simulink model "test3"  (Simulink 7.1)
settings: Solver=ode45  StartTime=0.0  StopTime=10.0  RelTol=1e-3
values from neighbouring files (symbols this model uses):
  Ctorque = cq(2:5:102,2:5:182)    [cq_table.m]
settings Model: Creator=xc  LastModifiedBy=xc

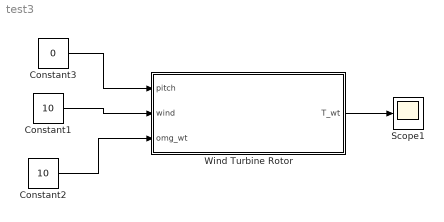
== system test3 ==
  Constant1 : Constant  Value=10  OutDataType=sfix(16)  OutScaling=2^0
  Constant2 : Constant  Value=10  OutDataType=sfix(16)  OutScaling=2^0
  Constant3 : Constant  Value=0  OutDataType=sfix(16)  OutScaling=2^0
  Scope1 : Scope
      settings: YMin=-2.25e+010  YMax=1.5e+010
  Wind Turbine Rotor : Subsystem  AncestorBlock=wt_blockset_beta/Mechanical Components/Wind Turbine Rotor  mask(Aerodynamic model for wind turbine){R=40, ro_air=1.25, cut_in=3, cut_out=25, Tact=1}
      mask prompts: R "Blade radius [m]"; ro_air "Air density [kg m3]"; cut_in "Cut in speed [m/sec]"; cut_out "Cut out speed [m/sec]"; Tact "Time constant for pitch actuator [sec]"
      mask init:
      | cq_table
      mask Display: plot(20,0,120,200,[45,35,35,45,75,75,45],[85,92,108,115,115,85,85],[55,50,70,65],[115,180,190,115],[55,50,70,65],[85,10,20,85],[75,85],[102,102],[75,85],[98,98],[105,85,85,105],[80,85,115,120])
  wires:
  Constant3/1 -> Wind Turbine Rotor/1(pitch)
  Constant1/1 -> Wind Turbine Rotor/2(wind)
  Constant2/1 -> Wind Turbine Rotor/3(omg_wt)
  Wind Turbine Rotor/1(T_wt) -> Scope1/1

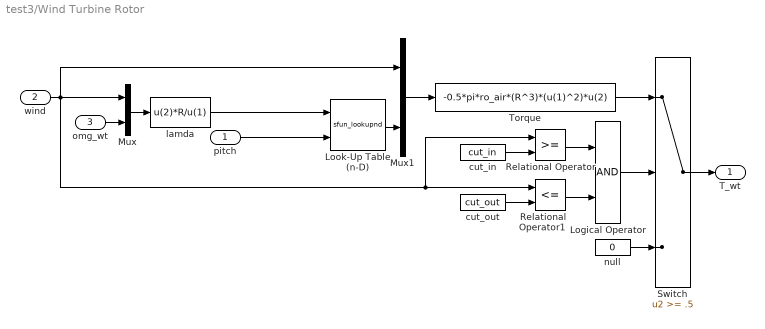
== system test3/Wind Turbine Rotor ==
  pitch : Inport  OutDataType=sfix(16)  OutScaling=2^0
  wind : Inport  Port=2  OutDataType=sfix(16)  OutScaling=2^0
  omg_wt : Inport  Port=3  OutDataType=sfix(16)  OutScaling=2^0
  Logical Operator : Logic
  Look-Up Table (n-D) : S-Function  FunctionName=sfun_lookupnd  Parameters=numDims,tableData,bp1,bp2,bp3,bp4,bpcell,searchMode,cacheBpFlag,vectorInputFlag,interpMethod,extrapMethod,rangeErrorMode  EnableBusSupport=off  mask(LookupNDInterp){numDimsPopupSelect=2, bp1=[0:1:20], bp2=[-90:5:90], bp3=[1:3], bp4=[1:3], bpcell={ [1:3], [1:3] }, explicitNumDims=2, searchMode=Binary Search, cacheBpFlag=off, vectorInputFlag=off, tableData=Ctorque, interpMethod=Linear, extrapMethod=None - Clip, rangeErrorMode=Error}
      mask prompts: numDimsPopupSelect "Number of table dimensions:"; bp1 "First input (row) breakpoint set:"; bp2 "Second (column) input breakpoint set:"; bp3 "Third input breakpoint set:"; bp4 "Fourth input breakpoint set:"; bpcell "Fifth..Nth breakpoint sets (cell array):"; explicitNumDims "Explicit number of dimensions:"; searchMode "Index search method:"; cacheBpFlag "Begin index searches using previous index results"; vectorInputFlag "Use one (vector) input port instead of N ports"; tableData "Table data:"; interpMethod "Interpolation method:"; extrapMethod "Extrapolation method:"; rangeErrorMode "Action for out of range input:"
      mask help: Perform n-dimensional interpolated table lookup including index searches. The table is a sampled representation of a function in N variables. Breakpoint sets relate the input values to positions in the table. The first dimension corresponds to the top (or left) input port.
      mask init:
      | if numDimsPopupSelect==5
      |   numDims=explicitNumDims;
      | else
      |   numDims=numDimsPopupSelect;
      | end
      | if strcmp(get_param(bdroot(gcb),'BlockDiagramType'),'library')
      |   dimsChar = 'n';
      | else
      |   dimsChar = sprintf('%d',numDims);
      | end
      | switch interpMethod
      |   case 1
      |     plottype = 'flatplot';
      |   case 2
      |     plottype = 'lineplot';
      |   otherwise
      |     plottype = 'splineplot';
      | end
      | for i=1:numDims
      |   switch( i )
      |     case 1
      |       bp = bp1;
      |     case 2
      |       bp = bp2;
      |     case 3
      |       bp = bp3;
      |     case 4
      |       bp = bp4;
      |     otherwise
      |       bp = bpcell{i-4};
      |    end
      |    Lbp = length(bp);
      |    if i < 2
      |      bpData = reshape(bp,Lbp,1);
      |      bpIndices = 0;
      |    else
      |      bpData = [ bpData; reshape(bp,Lbp,1) ];
      |      bpIndices = [ bpIndices; bpIndices(i-1)+LbpPrev ];
      |    end
      |    LbpPrev = Lbp;
      | end
      | [x,y,xaxes,yaxes] = ndlookico(plottype, numDims,{bpData,bpIndices,tableData});
      mask StyleString: popup(   1   |   2   |   3   |   4   |More...),edit,edit,edit,edit,edit,edit,popup(Evenly Spaced Points|Linear Search|Binary Search),checkbox,checkbox,edit,popup(None - Flat|Linear|Cubic Spline),popup(None - Clip|Linear|Cubic Spline),popup(None|Warning|Error)
      mask CallbackString: ndlookico|||||||||||||
      mask Display:
      | text(0.5,0.9,sprintf(' %s-D T(u)',dimsChar),'horizontalAlignment','center')
      | plot(x,y)
      | plot(xaxes,yaxes)
  Mux : Mux  Inputs=2
  Mux1 : Mux  Inputs=2
  Relational Operator : RelationalOperator  InputSameDT=on
  Relational Operator1 : RelationalOperator  Operator=<=  InputSameDT=on
  Switch : Switch  Threshold=.5  SaturateOnIntegerOverflow=on  InputSameDT=on
  Torque : Fcn  Expr=-0.5*pi*ro_air*(R^3)*(u(1)^2)*u(2)
  cut_in : Constant  Value=cut_in  OutDataType=sfix(16)  OutScaling=2^0
  cut_out : Constant  Value=cut_out  OutDataType=sfix(16)  OutScaling=2^0
  lamda : Fcn  Expr=u(2)*R/u(1)
  null : Constant  Value=0  OutDataType=sfix(16)  OutScaling=2^0
  T_wt : Outport
  wires:
  Mux/1 -> lamda/1
  Mux1/1 -> Torque/1
  omg_wt/1 -> Mux/2
  cut_in/1 -> Relational Operator/2
  cut_out/1 -> Relational Operator1/2
  Relational Operator1/1 -> Logical Operator/2
  Relational Operator/1 -> Logical Operator/1
  Switch/1 -> T_wt/1
  Torque/1 -> Switch/1
  null/1 -> Switch/3
  Logical Operator/1 -> Switch/2
  wind/1 -> Mux/1, Relational Operator/1, Relational Operator1/1, Mux1/1
  Look-Up Table (n-D)/1 -> Mux1/2
  lamda/1 -> Look-Up Table (n-D)/1
  pitch/1 -> Look-Up Table (n-D)/2
